simulink model "AMDSB"  (R2013b)
settings: Solver=ode45  StartTime=0.0  StopTime=10.0  RelTol=1e-3
libraries: dsparch4 x1
settings Model: Creator=Iqbal  LastModifiedBy=Iqbal

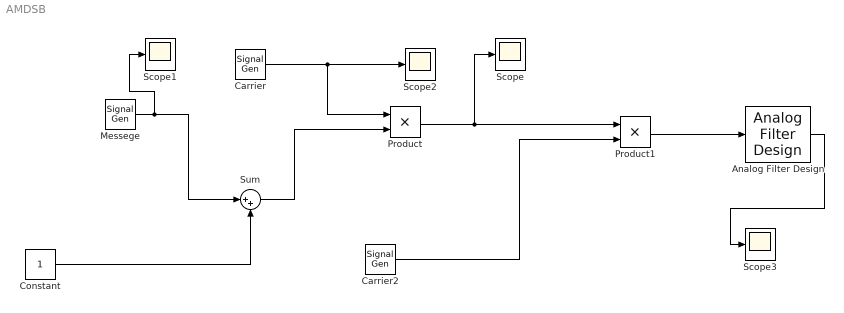
== system AMDSB ==
  Analog Filter Design : dsparch4/Analog Filter Design  method=Butterworth  filttype=Lowpass  N=8  Wlo=2*pi*2  Whi=80  Rp=2  Rs=40
  Carrier : SignalGenerator  Frequency=2*pi*10  Units=rad/sec
  Carrier2 : SignalGenerator  Frequency=2*pi*10  Units=rad/sec
  Constant : Constant
  Messege : SignalGenerator  Frequency=2*pi*2  Units=rad/sec
  Product : Product  SampleTime=0.01
  Product1 : Product  SampleTime=0.01
  Scope{,1..3} (4 alike) : Scope
      Scope2 settings: SaveName=ScopeData2
      Scope3 settings: SaveName=ScopeData3
  Sum : Sum  Inputs=|++
  wires:
  Messege/1 -> Scope1/1, Sum/1
  Constant/1 -> Sum/2
  Carrier/1 -> Product/1, Scope2/1
  Sum/1 -> Product/2
  Product/1 -> Scope/1, Product1/1
  Carrier2/1 -> Product1/2
  Product1/1 -> Analog Filter Design/1
  Analog Filter Design/1 -> Scope3/1
